simulink model "deep_bram"  (R2016b)
settings: Solver=VariableStepAuto  StartTime=0.0  StopTime=1000  RelTol=1e-3
libraries: xbsIndex_r4 x1049, casper_library_misc x1
(part 2 of 7)

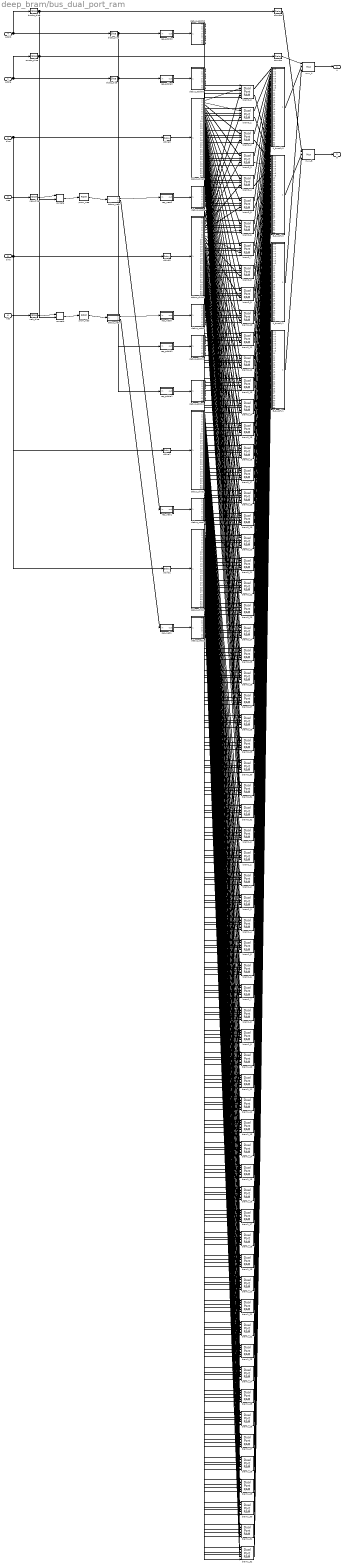
== system deep_bram/bus_dual_port_ram ==
  addra : Inport
  dina : Inport  Port=2
  wea : Inport  Port=3
  addrb : Inport  Port=4
  dinb : Inport  Port=5
  web : Inport  Port=6
  A_bussify0 : Subsystem  AncestorBlock=casper_library_flow_control/bus_create  mask(bus_create){inputNum=33}
      mask prompts: inputNum "Number of inputs:"
      mask init:
      | bus_create_init(gcb,...
      |     'inputNum', inputNum);
  A_bussify1 : Subsystem  AncestorBlock=casper_library_flow_control/bus_create  mask(bus_create){inputNum=33}
      mask prompts: inputNum "Number of inputs:"
      mask init:
      | bus_create_init(gcb,...
      |     'inputNum', inputNum);
  B_bussify0 : Subsystem  AncestorBlock=casper_library_flow_control/bus_create  mask(bus_create){inputNum=33}
      mask prompts: inputNum "Number of inputs:"
      mask init:
      | bus_create_init(gcb,...
      |     'inputNum', inputNum);
  B_bussify1 : Subsystem  AncestorBlock=casper_library_flow_control/bus_create  mask(bus_create){inputNum=33}
      mask prompts: inputNum "Number of inputs:"
      mask init:
      | bus_create_init(gcb,...
      |     'inputNum', inputNum);
  alsbs_slice : xbsIndex_r4/Slice  nbits=17  boolean_output=off  mode=Lower Bit Location + Width  bit1=0  base1=LSB of Input  bit0=0  base0=LSB of Input  dbl_ovrd=off  block_type=slice
  amsbs_slice : xbsIndex_r4/Slice  nbits=1  boolean_output=off  mode=Upper Bit Location + Width  bit1=0  base1=MSB of Input  bit0=0  base0=LSB of Input  dbl_ovrd=off  block_type=slice
  blsbs_slice : xbsIndex_r4/Slice  nbits=14  boolean_output=off  mode=Lower Bit Location + Width  bit1=0  base1=LSB of Input  bit0=0  base0=LSB of Input  dbl_ovrd=off  block_type=slice
  bmsbs_slice : xbsIndex_r4/Slice  nbits=1  boolean_output=off  mode=Upper Bit Location + Width  bit1=0  base1=MSB of Input  bit0=0  base0=LSB of Input  dbl_ovrd=off  block_type=slice
  bram0_{0..32} (33 alike) : xbsIndex_r4/Dual Port RAM  depth=131072  initVector=getfield(get_param(gcb, 'UserData'), 'initVector')  distributed_mem=Block RAM  init_a=0  init_b=0  rst_a=off  rst_b=off  en_a=off  en_b=off  latency=3  write_mode_A=Read Before Write  write_mode_B=Read Before Write  optimize=Speed  dbl_ovrd=off  block_type=dpram
  bram1_{0..32} (33 alike) : xbsIndex_r4/Dual Port RAM  depth=131072  initVector=getfield(get_param(gcb, 'UserData'), 'initVector')  distributed_mem=Block RAM  init_a=0  init_b=0  rst_a=off  rst_b=off  en_a=off  en_b=off  latency=3  write_mode_A=Read Before Write  write_mode_B=Read Before Write  optimize=Speed  dbl_ovrd=off  block_type=dpram
  concata : xbsIndex_r4/Concat  num_inputs=2  dbl_ovrd=off  block_type=concat
  concatb : xbsIndex_r4/Concat  num_inputs=2  dbl_ovrd=off  block_type=concat
  damsbs : xbsIndex_r4/Delay  rst=off  infoeditControl=Selection of Reset will increase slice count due to use of real FFs and instead of SRLs  en=off  latency=2+3  reg_retiming=off  dbl_ovrd=off  block_type=delay
      settings: infoedit=Hardware notes: A delay line is a chain, each link of which is an SRL16 or SRL32 followed by a flip-flop.
  dbmsbs : xbsIndex_r4/Delay  rst=off  infoeditControl=Selection of Reset will increase slice count due to use of real FFs and instead of SRLs  en=off  latency=2+3  reg_retiming=off  dbl_ovrd=off  block_type=delay
      settings: infoedit=Hardware notes: A delay line is a chain, each link of which is an SRL16 or SRL32 followed by a flip-flop.
  ddina0 : xbsIndex_r4/Delay  rst=off  infoeditControl=Selection of Reset will increase slice count due to use of real FFs and instead of SRLs  en=off  latency=2  reg_retiming=off  dbl_ovrd=off  block_type=delay
      settings: infoedit=Hardware notes: A delay line is a chain, each link of which is an SRL16 or SRL32 followed by a flip-flop.
  ddina1 : xbsIndex_r4/Delay  rst=off  infoeditControl=Selection of Reset will increase slice count due to use of real FFs and instead of SRLs  en=off  latency=2  reg_retiming=off  dbl_ovrd=off  block_type=delay
      settings: infoedit=Hardware notes: A delay line is a chain, each link of which is an SRL16 or SRL32 followed by a flip-flop.
  ddinb0 : xbsIndex_r4/Delay  rst=off  infoeditControl=Selection of Reset will increase slice count due to use of real FFs and instead of SRLs  en=off  latency=2  reg_retiming=off  dbl_ovrd=off  block_type=delay
      settings: infoedit=Hardware notes: A delay line is a chain, each link of which is an SRL16 or SRL32 followed by a flip-flop.
  ddinb1 : xbsIndex_r4/Delay  rst=off  infoeditControl=Selection of Reset will increase slice count due to use of real FFs and instead of SRLs  en=off  latency=2  reg_retiming=off  dbl_ovrd=off  block_type=delay
      settings: infoedit=Hardware notes: A delay line is a chain, each link of which is an SRL16 or SRL32 followed by a flip-flop.
  debus_addra0 : Subsystem  AncestorBlock=casper_library_flow_control/bus_expand  mask(bus_expand){mode=divisions of equal size, outputNum=9, outputWidth=[17 17 17 17 17 17 17 17 17], outputBinaryPt=[0 0 0 0 0 0 0 0 0], outputArithmeticType=[0 0 0 0 0 0 0 0 0], show_format=on, outputToWorkspace=off, variablePrefix=, outputToModelAsWell=on}
      mask prompts: outputNum "Number of outputs:"; outputWidth "Output width:"; outputBinaryPt "Output binary point position:"; outputArithmeticType "Output arithmetic type (ufix=0, fix=1, bool=2):"; show_format "Print format string?"; outputToWorkspace "Output to workspace?"; variablePrefix "Variable name prefix:"; outputToModelAsWell "Output to model as well?"
      mask help:
      | Expands a 'bus' made using a bus_create or Xilinx
      | concat block.
      | The input will be divided into the specified number
      | of outputs with the specified arithmetic types.
      | Divisions are made from most significant bit.
      mask init: same as deep_bram/bus_expand
      settings: AttributesFormatString=9 outputs: uf17.0,uf17.0,uf17.0,uf17.0,uf17.0,uf17.0,uf17.0,uf17.0,uf17.0,
      mask TypeOptions mode: divisions of equal size | divisions of arbitrary size
      mask Callback mode: bus_expand_callback();
      mask Callback outputWidth: bus_expand_callback();
      mask Callback outputToWorkspace: bus_expand_callback();
  debus_addra1 : Subsystem  AncestorBlock=casper_library_flow_control/bus_expand  mask(bus_expand){mode=divisions of equal size, outputNum=9, outputWidth=[17 17 17 17 17 17 17 17 17], outputBinaryPt=[0 0 0 0 0 0 0 0 0], outputArithmeticType=[0 0 0 0 0 0 0 0 0], show_format=on, outputToWorkspace=off, variablePrefix=, outputToModelAsWell=on}
      mask prompts: outputNum "Number of outputs:"; outputWidth "Output width:"; outputBinaryPt "Output binary point position:"; outputArithmeticType "Output arithmetic type (ufix=0, fix=1, bool=2):"; show_format "Print format string?"; outputToWorkspace "Output to workspace?"; variablePrefix "Variable name prefix:"; outputToModelAsWell "Output to model as well?"
      mask help:
      | Expands a 'bus' made using a bus_create or Xilinx
      | concat block.
      | The input will be divided into the specified number
      | of outputs with the specified arithmetic types.
      | Divisions are made from most significant bit.
      mask init: same as deep_bram/bus_expand
      settings: AttributesFormatString=9 outputs: uf17.0,uf17.0,uf17.0,uf17.0,uf17.0,uf17.0,uf17.0,uf17.0,uf17.0,
      mask TypeOptions mode: divisions of equal size | divisions of arbitrary size
      mask Callback mode: bus_expand_callback();
      mask Callback outputWidth: bus_expand_callback();
      mask Callback outputToWorkspace: bus_expand_callback();
  debus_addrb0 : Subsystem  AncestorBlock=casper_library_flow_control/bus_expand  mask(bus_expand){mode=divisions of equal size, outputNum=9, outputWidth=[14 14 14 14 14 14 14 14 14], outputBinaryPt=[0 0 0 0 0 0 0 0 0], outputArithmeticType=[0 0 0 0 0 0 0 0 0], show_format=on, outputToWorkspace=off, variablePrefix=, outputToModelAsWell=on}
      mask prompts: outputNum "Number of outputs:"; outputWidth "Output width:"; outputBinaryPt "Output binary point position:"; outputArithmeticType "Output arithmetic type (ufix=0, fix=1, bool=2):"; show_format "Print format string?"; outputToWorkspace "Output to workspace?"; variablePrefix "Variable name prefix:"; outputToModelAsWell "Output to model as well?"
      mask help:
      | Expands a 'bus' made using a bus_create or Xilinx
      | concat block.
      | The input will be divided into the specified number
      | of outputs with the specified arithmetic types.
      | Divisions are made from most significant bit.
      mask init: same as deep_bram/bus_expand
      settings: AttributesFormatString=9 outputs: uf14.0,uf14.0,uf14.0,uf14.0,uf14.0,uf14.0,uf14.0,uf14.0,uf14.0,
      mask TypeOptions mode: divisions of equal size | divisions of arbitrary size
      mask Callback mode: bus_expand_callback();
      mask Callback outputWidth: bus_expand_callback();
      mask Callback outputToWorkspace: bus_expand_callback();
  debus_addrb1 : Subsystem  AncestorBlock=casper_library_flow_control/bus_expand  mask(bus_expand){mode=divisions of equal size, outputNum=9, outputWidth=[14 14 14 14 14 14 14 14 14], outputBinaryPt=[0 0 0 0 0 0 0 0 0], outputArithmeticType=[0 0 0 0 0 0 0 0 0], show_format=on, outputToWorkspace=off, variablePrefix=, outputToModelAsWell=on}
      mask prompts: outputNum "Number of outputs:"; outputWidth "Output width:"; outputBinaryPt "Output binary point position:"; outputArithmeticType "Output arithmetic type (ufix=0, fix=1, bool=2):"; show_format "Print format string?"; outputToWorkspace "Output to workspace?"; variablePrefix "Variable name prefix:"; outputToModelAsWell "Output to model as well?"
      mask help:
      | Expands a 'bus' made using a bus_create or Xilinx
      | concat block.
      | The input will be divided into the specified number
      | of outputs with the specified arithmetic types.
      | Divisions are made from most significant bit.
      mask init: same as deep_bram/bus_expand
      settings: AttributesFormatString=9 outputs: uf14.0,uf14.0,uf14.0,uf14.0,uf14.0,uf14.0,uf14.0,uf14.0,uf14.0,
      mask TypeOptions mode: divisions of equal size | divisions of arbitrary size
      mask Callback mode: bus_expand_callback();
      mask Callback outputWidth: bus_expand_callback();
      mask Callback outputToWorkspace: bus_expand_callback();
  debus_dina0 : Subsystem  AncestorBlock=casper_library_flow_control/bus_expand  mask(bus_expand){mode=divisions of arbitrary size, outputNum=1, outputWidth=[1 1 1 1 1 1 1 1 1 1 1 1 1 1 1 1 1 1 1 1 1 1 1 1 1 1 1 1 1 1 1 1 1], outputBinaryPt=[0 0 0 0 0 0 0 0 0 0 0 0 0 0 0 0 0 0 0 0 0 0 0 0 0 0 0 0 0 0 0 0 0], outputArithmeticType=[0 0 0 0 0 0 0 0 0 0 0 0 0 0 0 0 0 0 0 0 0 0 0 0 0 0 0 0 0 0 0 0 0], show_format=on, outputToWorkspace=off, variablePrefix=, outputToModelAsWell=on}
      mask prompts: outputNum "Number of outputs:"; outputWidth "Output width [msb ... lsb]:"; outputBinaryPt "Output binary point position [msb ... lsb]:"; outputArithmeticType "Output arithmetic type (ufix=0, fix=1, bool=2) [msb ... lsb]:"; show_format "Print format string?"; outputToWorkspace "Output to workspace?"; variablePrefix "Variable name prefix:"; outputToModelAsWell "Output to model as well?"
      mask help:
      | Expands a 'bus' made using a bus_create or Xilinx
      | concat block.
      | The input will be divided into the specified number
      | of outputs with the specified arithmetic types.
      | Divisions are made from most significant bit.
      mask init: same as deep_bram/bus_expand
      settings: AttributesFormatString=33 outputs: uf1.0,uf1.0,uf1.0,uf1.0,uf1.0,uf1.0,uf1.0,uf1.0,uf1.0,uf1.0,uf1.0,uf1.0,uf1.0,uf1.0,uf1.0,uf1.0,uf1.0,uf1.0,uf1.0,uf1.0,uf1.0,uf1.0,uf1.0,uf1.0,uf1.0,uf1.0,uf1.0,uf1.0,uf1.0,uf1.0,uf1.0,uf1.0,uf1.0,
      mask TypeOptions mode: divisions of equal size | divisions of arbitrary size
      mask Callback mode: bus_expand_callback();
      mask Callback outputWidth: bus_expand_callback();
      mask Callback outputToWorkspace: bus_expand_callback();
  debus_dina1 : Subsystem  AncestorBlock=casper_library_flow_control/bus_expand  mask(bus_expand){mode=divisions of arbitrary size, outputNum=1, outputWidth=[1 1 1 1 1 1 1 1 1 1 1 1 1 1 1 1 1 1 1 1 1 1 1 1 1 1 1 1 1 1 1 1 1], outputBinaryPt=[0 0 0 0 0 0 0 0 0 0 0 0 0 0 0 0 0 0 0 0 0 0 0 0 0 0 0 0 0 0 0 0 0], outputArithmeticType=[0 0 0 0 0 0 0 0 0 0 0 0 0 0 0 0 0 0 0 0 0 0 0 0 0 0 0 0 0 0 0 0 0], show_format=on, outputToWorkspace=off, variablePrefix=, outputToModelAsWell=on}
      mask prompts: outputNum "Number of outputs:"; outputWidth "Output width [msb ... lsb]:"; outputBinaryPt "Output binary point position [msb ... lsb]:"; outputArithmeticType "Output arithmetic type (ufix=0, fix=1, bool=2) [msb ... lsb]:"; show_format "Print format string?"; outputToWorkspace "Output to workspace?"; variablePrefix "Variable name prefix:"; outputToModelAsWell "Output to model as well?"
      mask help:
      | Expands a 'bus' made using a bus_create or Xilinx
      | concat block.
      | The input will be divided into the specified number
      | of outputs with the specified arithmetic types.
      | Divisions are made from most significant bit.
      mask init: same as deep_bram/bus_expand
      settings: AttributesFormatString=33 outputs: uf1.0,uf1.0,uf1.0,uf1.0,uf1.0,uf1.0,uf1.0,uf1.0,uf1.0,uf1.0,uf1.0,uf1.0,uf1.0,uf1.0,uf1.0,uf1.0,uf1.0,uf1.0,uf1.0,uf1.0,uf1.0,uf1.0,uf1.0,uf1.0,uf1.0,uf1.0,uf1.0,uf1.0,uf1.0,uf1.0,uf1.0,uf1.0,uf1.0,
      mask TypeOptions mode: divisions of equal size | divisions of arbitrary size
      mask Callback mode: bus_expand_callback();
      mask Callback outputWidth: bus_expand_callback();
      mask Callback outputToWorkspace: bus_expand_callback();
  debus_dinb0 : Subsystem  AncestorBlock=casper_library_flow_control/bus_expand  mask(bus_expand){mode=divisions of arbitrary size, outputNum=1, outputWidth=[8 8 8 8 8 8 8 8 8 8 8 8 8 8 8 8 8 8 8 8 8 8 8 8 8 8 8 8 8 8 8 8 8], outputBinaryPt=[0 0 0 0 0 0 0 0 0 0 0 0 0 0 0 0 0 0 0 0 0 0 0 0 0 0 0 0 0 0 0 0 0], outputArithmeticType=[0 0 0 0 0 0 0 0 0 0 0 0 0 0 0 0 0 0 0 0 0 0 0 0 0 0 0 0 0 0 0 0 0], show_format=on, outputToWorkspace=off, variablePrefix=, outputToModelAsWell=on}
      mask prompts: outputNum "Number of outputs:"; outputWidth "Output width [msb ... lsb]:"; outputBinaryPt "Output binary point position [msb ... lsb]:"; outputArithmeticType "Output arithmetic type (ufix=0, fix=1, bool=2) [msb ... lsb]:"; show_format "Print format string?"; outputToWorkspace "Output to workspace?"; variablePrefix "Variable name prefix:"; outputToModelAsWell "Output to model as well?"
      mask help:
      | Expands a 'bus' made using a bus_create or Xilinx
      | concat block.
      | The input will be divided into the specified number
      | of outputs with the specified arithmetic types.
      | Divisions are made from most significant bit.
      mask init: same as deep_bram/bus_expand
      settings: AttributesFormatString=33 outputs: uf8.0,uf8.0,uf8.0,uf8.0,uf8.0,uf8.0,uf8.0,uf8.0,uf8.0,uf8.0,uf8.0,uf8.0,uf8.0,uf8.0,uf8.0,uf8.0,uf8.0,uf8.0,uf8.0,uf8.0,uf8.0,uf8.0,uf8.0,uf8.0,uf8.0,uf8.0,uf8.0,uf8.0,uf8.0,uf8.0,uf8.0,uf8.0,uf8.0,
      mask TypeOptions mode: divisions of equal size | divisions of arbitrary size
      mask Callback mode: bus_expand_callback();
      mask Callback outputWidth: bus_expand_callback();
      mask Callback outputToWorkspace: bus_expand_callback();
  debus_dinb1 : Subsystem  AncestorBlock=casper_library_flow_control/bus_expand  mask(bus_expand){mode=divisions of arbitrary size, outputNum=1, outputWidth=[8 8 8 8 8 8 8 8 8 8 8 8 8 8 8 8 8 8 8 8 8 8 8 8 8 8 8 8 8 8 8 8 8], outputBinaryPt=[0 0 0 0 0 0 0 0 0 0 0 0 0 0 0 0 0 0 0 0 0 0 0 0 0 0 0 0 0 0 0 0 0], outputArithmeticType=[0 0 0 0 0 0 0 0 0 0 0 0 0 0 0 0 0 0 0 0 0 0 0 0 0 0 0 0 0 0 0 0 0], show_format=on, outputToWorkspace=off, variablePrefix=, outputToModelAsWell=on}
      mask prompts: outputNum "Number of outputs:"; outputWidth "Output width [msb ... lsb]:"; outputBinaryPt "Output binary point position [msb ... lsb]:"; outputArithmeticType "Output arithmetic type (ufix=0, fix=1, bool=2) [msb ... lsb]:"; show_format "Print format string?"; outputToWorkspace "Output to workspace?"; variablePrefix "Variable name prefix:"; outputToModelAsWell "Output to model as well?"
      mask help:
      | Expands a 'bus' made using a bus_create or Xilinx
      | concat block.
      | The input will be divided into the specified number
      | of outputs with the specified arithmetic types.
      | Divisions are made from most significant bit.
      mask init: same as deep_bram/bus_expand
      settings: AttributesFormatString=33 outputs: uf8.0,uf8.0,uf8.0,uf8.0,uf8.0,uf8.0,uf8.0,uf8.0,uf8.0,uf8.0,uf8.0,uf8.0,uf8.0,uf8.0,uf8.0,uf8.0,uf8.0,uf8.0,uf8.0,uf8.0,uf8.0,uf8.0,uf8.0,uf8.0,uf8.0,uf8.0,uf8.0,uf8.0,uf8.0,uf8.0,uf8.0,uf8.0,uf8.0,
      mask TypeOptions mode: divisions of equal size | divisions of arbitrary size
      mask Callback mode: bus_expand_callback();
      mask Callback outputWidth: bus_expand_callback();
      mask Callback outputToWorkspace: bus_expand_callback();
  debus_wea : Subsystem  AncestorBlock=casper_library_flow_control/bus_expand  mask(bus_expand){mode=divisions of equal size, outputNum=2, outputWidth=[1 1], outputBinaryPt=[0 0], outputArithmeticType=[2 2], show_format=on, outputToWorkspace=off, variablePrefix=, outputToModelAsWell=on}
      mask prompts: outputNum "Number of outputs:"; outputWidth "Output width:"; outputBinaryPt "Output binary point position:"; outputArithmeticType "Output arithmetic type (ufix=0, fix=1, bool=2):"; show_format "Print format string?"; outputToWorkspace "Output to workspace?"; variablePrefix "Variable name prefix:"; outputToModelAsWell "Output to model as well?"
      mask help:
      | Expands a 'bus' made using a bus_create or Xilinx
      | concat block.
      | The input will be divided into the specified number
      | of outputs with the specified arithmetic types.
      | Divisions are made from most significant bit.
      mask init: same as deep_bram/bus_expand
      settings: AttributesFormatString=2 outputs: b,b,
      mask TypeOptions mode: divisions of equal size | divisions of arbitrary size
      mask Callback mode: bus_expand_callback();
      mask Callback outputWidth: bus_expand_callback();
      mask Callback outputToWorkspace: bus_expand_callback();
  debus_wea0 : Subsystem  AncestorBlock=casper_library_flow_control/bus_expand  mask(bus_expand){mode=divisions of equal size, outputNum=9, outputWidth=[1 1 1 1 1 1 1 1 1], outputBinaryPt=[0 0 0 0 0 0 0 0 0], outputArithmeticType=[2 2 2 2 2 2 2 2 2], show_format=on, outputToWorkspace=off, variablePrefix=, outputToModelAsWell=on}
      mask prompts: outputNum "Number of outputs:"; outputWidth "Output width:"; outputBinaryPt "Output binary point position:"; outputArithmeticType "Output arithmetic type (ufix=0, fix=1, bool=2):"; show_format "Print format string?"; outputToWorkspace "Output to workspace?"; variablePrefix "Variable name prefix:"; outputToModelAsWell "Output to model as well?"
      mask help:
      | Expands a 'bus' made using a bus_create or Xilinx
      | concat block.
      | The input will be divided into the specified number
      | of outputs with the specified arithmetic types.
      | Divisions are made from most significant bit.
      mask init: same as deep_bram/bus_expand
      settings: AttributesFormatString=9 outputs: b,b,b,b,b,b,b,b,b,
      mask TypeOptions mode: divisions of equal size | divisions of arbitrary size
      mask Callback mode: bus_expand_callback();
      mask Callback outputWidth: bus_expand_callback();
      mask Callback outputToWorkspace: bus_expand_callback();
  debus_wea1 : Subsystem  AncestorBlock=casper_library_flow_control/bus_expand  mask(bus_expand){mode=divisions of equal size, outputNum=9, outputWidth=[1 1 1 1 1 1 1 1 1], outputBinaryPt=[0 0 0 0 0 0 0 0 0], outputArithmeticType=[2 2 2 2 2 2 2 2 2], show_format=on, outputToWorkspace=off, variablePrefix=, outputToModelAsWell=on}
      mask prompts: outputNum "Number of outputs:"; outputWidth "Output width:"; outputBinaryPt "Output binary point position:"; outputArithmeticType "Output arithmetic type (ufix=0, fix=1, bool=2):"; show_format "Print format string?"; outputToWorkspace "Output to workspace?"; variablePrefix "Variable name prefix:"; outputToModelAsWell "Output to model as well?"
      mask help:
      | Expands a 'bus' made using a bus_create or Xilinx
      | concat block.
      | The input will be divided into the specified number
      | of outputs with the specified arithmetic types.
      | Divisions are made from most significant bit.
      mask init: same as deep_bram/bus_expand
      settings: AttributesFormatString=9 outputs: b,b,b,b,b,b,b,b,b,
      mask TypeOptions mode: divisions of equal size | divisions of arbitrary size
      mask Callback mode: bus_expand_callback();
      mask Callback outputWidth: bus_expand_callback();
      mask Callback outputToWorkspace: bus_expand_callback();
  debus_web : Subsystem  AncestorBlock=casper_library_flow_control/bus_expand  mask(bus_expand){mode=divisions of equal size, outputNum=2, outputWidth=[1 1], outputBinaryPt=[0 0], outputArithmeticType=[2 2], show_format=on, outputToWorkspace=off, variablePrefix=, outputToModelAsWell=on}
      mask prompts: outputNum "Number of outputs:"; outputWidth "Output width:"; outputBinaryPt "Output binary point position:"; outputArithmeticType "Output arithmetic type (ufix=0, fix=1, bool=2):"; show_format "Print format string?"; outputToWorkspace "Output to workspace?"; variablePrefix "Variable name prefix:"; outputToModelAsWell "Output to model as well?"
      mask help:
      | Expands a 'bus' made using a bus_create or Xilinx
      | concat block.
      | The input will be divided into the specified number
      | of outputs with the specified arithmetic types.
      | Divisions are made from most significant bit.
      mask init: same as deep_bram/bus_expand
      settings: AttributesFormatString=2 outputs: b,b,
      mask TypeOptions mode: divisions of equal size | divisions of arbitrary size
      mask Callback mode: bus_expand_callback();
      mask Callback outputWidth: bus_expand_callback();
      mask Callback outputToWorkspace: bus_expand_callback();
  debus_web0 : Subsystem  AncestorBlock=casper_library_flow_control/bus_expand  mask(bus_expand){mode=divisions of equal size, outputNum=9, outputWidth=[1 1 1 1 1 1 1 1 1], outputBinaryPt=[0 0 0 0 0 0 0 0 0], outputArithmeticType=[2 2 2 2 2 2 2 2 2], show_format=on, outputToWorkspace=off, variablePrefix=, outputToModelAsWell=on}
      mask prompts: outputNum "Number of outputs:"; outputWidth "Output width:"; outputBinaryPt "Output binary point position:"; outputArithmeticType "Output arithmetic type (ufix=0, fix=1, bool=2):"; show_format "Print format string?"; outputToWorkspace "Output to workspace?"; variablePrefix "Variable name prefix:"; outputToModelAsWell "Output to model as well?"
      mask help:
      | Expands a 'bus' made using a bus_create or Xilinx
      | concat block.
      | The input will be divided into the specified number
      | of outputs with the specified arithmetic types.
      | Divisions are made from most significant bit.
      mask init: same as deep_bram/bus_expand
      settings: AttributesFormatString=9 outputs: b,b,b,b,b,b,b,b,b,
      mask TypeOptions mode: divisions of equal size | divisions of arbitrary size
      mask Callback mode: bus_expand_callback();
      mask Callback outputWidth: bus_expand_callback();
      mask Callback outputToWorkspace: bus_expand_callback();
  debus_web1 : Subsystem  AncestorBlock=casper_library_flow_control/bus_expand  mask(bus_expand){mode=divisions of equal size, outputNum=9, outputWidth=[1 1 1 1 1 1 1 1 1], outputBinaryPt=[0 0 0 0 0 0 0 0 0], outputArithmeticType=[2 2 2 2 2 2 2 2 2], show_format=on, outputToWorkspace=off, variablePrefix=, outputToModelAsWell=on}
      mask prompts: outputNum "Number of outputs:"; outputWidth "Output width:"; outputBinaryPt "Output binary point position:"; outputArithmeticType "Output arithmetic type (ufix=0, fix=1, bool=2):"; show_format "Print format string?"; outputToWorkspace "Output to workspace?"; variablePrefix "Variable name prefix:"; outputToModelAsWell "Output to model as well?"
      mask help:
      | Expands a 'bus' made using a bus_create or Xilinx
      | concat block.
      | The input will be divided into the specified number
      | of outputs with the specified arithmetic types.
      | Divisions are made from most significant bit.
      mask init: same as deep_bram/bus_expand
      settings: AttributesFormatString=9 outputs: b,b,b,b,b,b,b,b,b,
      mask TypeOptions mode: divisions of equal size | divisions of arbitrary size
      mask Callback mode: bus_expand_callback();
      mask Callback outputWidth: bus_expand_callback();
      mask Callback outputToWorkspace: bus_expand_callback();
  mux_A : xbsIndex_r4/Mux  inputs=2  en=off  latency=0  precision=Full  arith_type=Unsigned  n_bits=16  bin_pt=14  quantization=Truncate  overflow=Wrap  dbl_ovrd=off  block_type=mux
  mux_B : xbsIndex_r4/Mux  inputs=2  en=off  latency=0  precision=Full  arith_type=Unsigned  n_bits=16  bin_pt=14  quantization=Truncate  overflow=Wrap  dbl_ovrd=off  block_type=mux
  prom_wea : xbsIndex_r4/ROM  depth=4  initVector=[0 0 2 1]  distributed_mem=Distributed memory  rst=off  init_reg=0  en=off  latency=0  gui_display_data_type=Fixed-point  arith_type=Unsigned  n_bits=2  bin_pt=0  preci_type=Single  exp_width=8  frac_width=24  optimize=Area  use_rpm=on  dbl_ovrd=off  block_type=sprom
  prom_web : xbsIndex_r4/ROM  depth=4  initVector=[0 0 2 1]  distributed_mem=Distributed memory  rst=off  init_reg=0  en=off  latency=0  gui_display_data_type=Fixed-point  arith_type=Unsigned  n_bits=2  bin_pt=0  preci_type=Single  exp_width=8  frac_width=24  optimize=Area  use_rpm=on  dbl_ovrd=off  block_type=sprom
  rep_addra0 : Subsystem  AncestorBlock=casper_library_bus/bus_replicate  mask(bus_replicate){replication=9, latency=2, misc=off, implementation=core}
      mask prompts: replication "replication factor"; misc "misc support"; implementation "delay implementation"
      mask help: Output bus formed by replicating input bus a number of times
      mask init:
      | bus_replicate_init(gcb, ...
      |     'replication', replication, ...
      |     'latency', latency, ...
      |     'implementation', implementation, ...
      |     'misc', misc);
      mask TypeOptions implementation: core | behavioral
  rep_addra1 : Subsystem  AncestorBlock=casper_library_bus/bus_replicate  mask(bus_replicate){replication=9, latency=2, misc=off, implementation=core}
      mask prompts: replication "replication factor"; misc "misc support"; implementation "delay implementation"
      mask help: Output bus formed by replicating input bus a number of times
      mask init:
      | bus_replicate_init(gcb, ...
      |     'replication', replication, ...
      |     'latency', latency, ...
      |     'implementation', implementation, ...
      |     'misc', misc);
      mask TypeOptions implementation: core | behavioral
  rep_addrb0 : Subsystem  AncestorBlock=casper_library_bus/bus_replicate  mask(bus_replicate){replication=9, latency=2, misc=off, implementation=core}
      mask prompts: replication "replication factor"; misc "misc support"; implementation "delay implementation"
      mask help: Output bus formed by replicating input bus a number of times
      mask init:
      | bus_replicate_init(gcb, ...
      |     'replication', replication, ...
      |     'latency', latency, ...
      |     'implementation', implementation, ...
      |     'misc', misc);
      mask TypeOptions implementation: core | behavioral
  rep_addrb1 : Subsystem  AncestorBlock=casper_library_bus/bus_replicate  mask(bus_replicate){replication=9, latency=2, misc=off, implementation=core}
      mask prompts: replication "replication factor"; misc "misc support"; implementation "delay implementation"
      mask help: Output bus formed by replicating input bus a number of times
      mask init:
      | bus_replicate_init(gcb, ...
      |     'replication', replication, ...
      |     'latency', latency, ...
      |     'implementation', implementation, ...
      |     'misc', misc);
      mask TypeOptions implementation: core | behavioral
  rep_wea0 : Subsystem  AncestorBlock=casper_library_bus/bus_replicate  mask(bus_replicate){replication=9, latency=2, misc=off, implementation=core}
      mask prompts: replication "replication factor"; misc "misc support"; implementation "delay implementation"
      mask help: Output bus formed by replicating input bus a number of times
      mask init:
      | bus_replicate_init(gcb, ...
      |     'replication', replication, ...
      |     'latency', latency, ...
      |     'implementation', implementation, ...
      |     'misc', misc);
      mask TypeOptions implementation: core | behavioral
  rep_wea1 : Subsystem  AncestorBlock=casper_library_bus/bus_replicate  mask(bus_replicate){replication=9, latency=2, misc=off, implementation=core}
      mask prompts: replication "replication factor"; misc "misc support"; implementation "delay implementation"
      mask help: Output bus formed by replicating input bus a number of times
      mask init:
      | bus_replicate_init(gcb, ...
      |     'replication', replication, ...
      |     'latency', latency, ...
      |     'implementation', implementation, ...
      |     'misc', misc);
      mask TypeOptions implementation: core | behavioral
  rep_web0 : Subsystem  AncestorBlock=casper_library_bus/bus_replicate  mask(bus_replicate){replication=9, latency=2, misc=off, implementation=core}
      mask prompts: replication "replication factor"; misc "misc support"; implementation "delay implementation"
      mask help: Output bus formed by replicating input bus a number of times
      mask init:
      | bus_replicate_init(gcb, ...
      |     'replication', replication, ...
      |     'latency', latency, ...
      |     'implementation', implementation, ...
      |     'misc', misc);
      mask TypeOptions implementation: core | behavioral
  rep_web1 : Subsystem  AncestorBlock=casper_library_bus/bus_replicate  mask(bus_replicate){replication=9, latency=2, misc=off, implementation=core}
      mask prompts: replication "replication factor"; misc "misc support"; implementation "delay implementation"
      mask help: Output bus formed by replicating input bus a number of times
      mask init:
      | bus_replicate_init(gcb, ...
      |     'replication', replication, ...
      |     'latency', latency, ...
      |     'implementation', implementation, ...
      |     'misc', misc);
      mask TypeOptions implementation: core | behavioral
  wea_slice : xbsIndex_r4/Slice  nbits=1  boolean_output=off  mode=Upper Bit Location + Width  bit1=0  base1=MSB of Input  bit0=0  base0=LSB of Input  dbl_ovrd=off  block_type=slice
  web_slice : xbsIndex_r4/Slice  nbits=1  boolean_output=off  mode=Upper Bit Location + Width  bit1=0  base1=MSB of Input  bit0=0  base0=LSB of Input  dbl_ovrd=off  block_type=slice
  A : Outport
  B : Outport  Port=2
  wires:
  addrb/1 -> bmsbs_slice/1, blsbs_slice/1
  addra/1 -> amsbs_slice/1, alsbs_slice/1
  wea/1 -> wea_slice/1
  web/1 -> web_slice/1
  wea_slice/1 -> concata/1
  amsbs_slice/1 -> concata/2, damsbs/1
  web_slice/1 -> concatb/1
  bmsbs_slice/1 -> concatb/2, dbmsbs/1
  concata/1 -> prom_wea/1
  concatb/1 -> prom_web/1
  prom_wea/1 -> debus_wea/1(bus_in)
  prom_web/1 -> debus_web/1(bus_in)
  blsbs_slice/1 -> rep_addrb0/1(in), rep_addrb1/1(in)
  alsbs_slice/1 -> rep_addra0/1(in), rep_addra1/1(in)
  dina/1 -> ddina0/1, ddina1/1
  debus_wea/1(msb_out2) -> rep_wea0/1(in)
  dinb/1 -> ddinb0/1, ddinb1/1
  debus_web/1(msb_out2) -> rep_web0/1(in)
  debus_wea/2(lsb_out1) -> rep_wea1/1(in)
  debus_web/2(lsb_out1) -> rep_web1/1(in)
  rep_addrb0/1(out) -> debus_addrb0/1(bus_in)
  rep_addra0/1(out) -> debus_addra0/1(bus_in)
  ddina0/1 -> debus_dina0/1(bus_in)
  rep_wea0/1(out) -> debus_wea0/1(bus_in)
  ddinb0/1 -> debus_dinb0/1(bus_in)
  rep_web0/1(out) -> debus_web0/1(bus_in)
  rep_addrb1/1(out) -> debus_addrb1/1(bus_in)
  rep_addra1/1(out) -> debus_addra1/1(bus_in)
  ddina1/1 -> debus_dina1/1(bus_in)
  rep_wea1/1(out) -> debus_wea1/1(bus_in)
  ddinb1/1 -> debus_dinb1/1(bus_in)
  rep_web1/1(out) -> debus_web1/1(bus_in)
  debus_addra0/1(msb_out9) -> bram0_0/1, bram0_9/1, bram0_18/1, bram0_27/1
  debus_dina0/1(msb_out33) -> bram0_0/2
  debus_wea0/1(msb_out9) -> bram0_0/3, bram0_9/3, bram0_18/3, bram0_27/3
  debus_addrb0/1(msb_out9) -> bram0_0/4, bram0_9/4, bram0_18/4, bram0_27/4
  debus_dinb0/1(msb_out33) -> bram0_0/5
  debus_web0/1(msb_out9) -> bram0_0/6, bram0_9/6, bram0_18/6, bram0_27/6
  debus_addra0/2(out8) -> bram0_1/1, bram0_10/1, bram0_19/1, bram0_28/1
  debus_dina0/2(out32) -> bram0_1/2
  debus_wea0/2(out8) -> bram0_1/3, bram0_10/3, bram0_19/3, bram0_28/3
  debus_addrb0/2(out8) -> bram0_1/4, bram0_10/4, bram0_19/4, bram0_28/4
  debus_dinb0/2(out32) -> bram0_1/5
  debus_web0/2(out8) -> bram0_1/6, bram0_10/6, bram0_19/6, bram0_28/6
  debus_addra0/3(out7) -> bram0_2/1, bram0_11/1, bram0_20/1, bram0_29/1
  debus_dina0/3(out31) -> bram0_2/2
  debus_wea0/3(out7) -> bram0_2/3, bram0_11/3, bram0_20/3, bram0_29/3
  debus_addrb0/3(out7) -> bram0_2/4, bram0_11/4, bram0_20/4, bram0_29/4
  debus_dinb0/3(out31) -> bram0_2/5
  debus_web0/3(out7) -> bram0_2/6, bram0_11/6, bram0_20/6, bram0_29/6
  debus_addra0/4(out6) -> bram0_3/1, bram0_12/1, bram0_21/1, bram0_30/1
  debus_dina0/4(out30) -> bram0_3/2
  debus_wea0/4(out6) -> bram0_3/3, bram0_12/3, bram0_21/3, bram0_30/3
  debus_addrb0/4(out6) -> bram0_3/4, bram0_12/4, bram0_21/4, bram0_30/4
  debus_dinb0/4(out30) -> bram0_3/5
  debus_web0/4(out6) -> bram0_3/6, bram0_12/6, bram0_21/6, bram0_30/6
  debus_addra0/5(out5) -> bram0_4/1, bram0_13/1, bram0_22/1, bram0_31/1
  debus_dina0/5(out29) -> bram0_4/2
  debus_wea0/5(out5) -> bram0_4/3, bram0_13/3, bram0_22/3, bram0_31/3
  debus_addrb0/5(out5) -> bram0_4/4, bram0_13/4, bram0_22/4, bram0_31/4
  debus_dinb0/5(out29) -> bram0_4/5
  debus_web0/5(out5) -> bram0_4/6, bram0_13/6, bram0_22/6, bram0_31/6
  debus_addra0/6(out4) -> bram0_5/1, bram0_14/1, bram0_23/1, bram0_32/1
  debus_dina0/6(out28) -> bram0_5/2
  debus_wea0/6(out4) -> bram0_5/3, bram0_14/3, bram0_23/3, bram0_32/3
  debus_addrb0/6(out4) -> bram0_5/4, bram0_14/4, bram0_23/4, bram0_32/4
  debus_dinb0/6(out28) -> bram0_5/5
  debus_web0/6(out4) -> bram0_5/6, bram0_14/6, bram0_23/6, bram0_32/6
  debus_addra0/7(out3) -> bram0_6/1, bram0_15/1, bram0_24/1
  debus_dina0/7(out27) -> bram0_6/2
  debus_wea0/7(out3) -> bram0_6/3, bram0_15/3, bram0_24/3
  debus_addrb0/7(out3) -> bram0_6/4, bram0_15/4, bram0_24/4
  debus_dinb0/7(out27) -> bram0_6/5
  debus_web0/7(out3) -> bram0_6/6, bram0_15/6, bram0_24/6
  debus_addra0/8(out2) -> bram0_7/1, bram0_16/1, bram0_25/1
  debus_dina0/8(out26) -> bram0_7/2
  debus_wea0/8(out2) -> bram0_7/3, bram0_16/3, bram0_25/3
  debus_addrb0/8(out2) -> bram0_7/4, bram0_16/4, bram0_25/4
  debus_dinb0/8(out26) -> bram0_7/5
  debus_web0/8(out2) -> bram0_7/6, bram0_16/6, bram0_25/6
  debus_addra0/9(lsb_out1) -> bram0_8/1, bram0_17/1, bram0_26/1
  debus_dina0/9(out25) -> bram0_8/2
  debus_wea0/9(lsb_out1) -> bram0_8/3, bram0_17/3, bram0_26/3
  debus_addrb0/9(lsb_out1) -> bram0_8/4, bram0_17/4, bram0_26/4
  debus_dinb0/9(out25) -> bram0_8/5
  debus_web0/9(lsb_out1) -> bram0_8/6, bram0_17/6, bram0_26/6
  debus_dina0/10(out24) -> bram0_9/2
  debus_dinb0/10(out24) -> bram0_9/5
  debus_dina0/11(out23) -> bram0_10/2
  debus_dinb0/11(out23) -> bram0_10/5
  debus_dina0/12(out22) -> bram0_11/2
  debus_dinb0/12(out22) -> bram0_11/5
  debus_dina0/13(out21) -> bram0_12/2
  debus_dinb0/13(out21) -> bram0_12/5
  debus_dina0/14(out20) -> bram0_13/2
  debus_dinb0/14(out20) -> bram0_13/5
  debus_dina0/15(out19) -> bram0_14/2
  debus_dinb0/15(out19) -> bram0_14/5
  debus_dina0/16(out18) -> bram0_15/2
  debus_dinb0/16(out18) -> bram0_15/5
  debus_dina0/17(out17) -> bram0_16/2
  debus_dinb0/17(out17) -> bram0_16/5
  debus_dina0/18(out16) -> bram0_17/2
  debus_dinb0/18(out16) -> bram0_17/5
  debus_dina0/19(out15) -> bram0_18/2
  debus_dinb0/19(out15) -> bram0_18/5
  debus_dina0/20(out14) -> bram0_19/2
  debus_dinb0/20(out14) -> bram0_19/5
  debus_dina0/21(out13) -> bram0_20/2
  debus_dinb0/21(out13) -> bram0_20/5
  debus_dina0/22(out12) -> bram0_21/2
  debus_dinb0/22(out12) -> bram0_21/5
  debus_dina0/23(out11) -> bram0_22/2
  debus_dinb0/23(out11) -> bram0_22/5
  debus_dina0/24(out10) -> bram0_23/2
  debus_dinb0/24(out10) -> bram0_23/5
  debus_dina0/25(out9) -> bram0_24/2
  debus_dinb0/25(out9) -> bram0_24/5
  debus_dina0/26(out8) -> bram0_25/2
  debus_dinb0/26(out8) -> bram0_25/5
  debus_dina0/27(out7) -> bram0_26/2
  debus_dinb0/27(out7) -> bram0_26/5
  debus_dina0/28(out6) -> bram0_27/2
  debus_dinb0/28(out6) -> bram0_27/5
  debus_dina0/29(out5) -> bram0_28/2
  debus_dinb0/29(out5) -> bram0_28/5
  debus_dina0/30(out4) -> bram0_29/2
  debus_dinb0/30(out4) -> bram0_29/5
  debus_dina0/31(out3) -> bram0_30/2
  debus_dinb0/31(out3) -> bram0_30/5
  debus_dina0/32(out2) -> bram0_31/2
  debus_dinb0/32(out2) -> bram0_31/5
  debus_dina0/33(lsb_out1) -> bram0_32/2
  debus_dinb0/33(lsb_out1) -> bram0_32/5
  debus_addra1/1(msb_out9) -> bram1_0/1, bram1_9/1, bram1_18/1, bram1_27/1
  debus_dina1/1(msb_out33) -> bram1_0/2
  debus_wea1/1(msb_out9) -> bram1_0/3, bram1_9/3, bram1_18/3, bram1_27/3
  debus_addrb1/1(msb_out9) -> bram1_0/4, bram1_9/4, bram1_18/4, bram1_27/4
  debus_dinb1/1(msb_out33) -> bram1_0/5
  debus_web1/1(msb_out9) -> bram1_0/6, bram1_9/6, bram1_18/6, bram1_27/6
  debus_addra1/2(out8) -> bram1_1/1, bram1_10/1, bram1_19/1, bram1_28/1
  debus_dina1/2(out32) -> bram1_1/2
  debus_wea1/2(out8) -> bram1_1/3, bram1_10/3, bram1_19/3, bram1_28/3
  debus_addrb1/2(out8) -> bram1_1/4, bram1_10/4, bram1_19/4, bram1_28/4
  debus_dinb1/2(out32) -> bram1_1/5
  debus_web1/2(out8) -> bram1_1/6, bram1_10/6, bram1_19/6, bram1_28/6
  debus_addra1/3(out7) -> bram1_2/1, bram1_11/1, bram1_20/1, bram1_29/1
  debus_dina1/3(out31) -> bram1_2/2
  debus_wea1/3(out7) -> bram1_2/3, bram1_11/3, bram1_20/3, bram1_29/3
  debus_addrb1/3(out7) -> bram1_2/4, bram1_11/4, bram1_20/4, bram1_29/4
  debus_dinb1/3(out31) -> bram1_2/5
  debus_web1/3(out7) -> bram1_2/6, bram1_11/6, bram1_20/6, bram1_29/6
  debus_addra1/4(out6) -> bram1_3/1, bram1_12/1, bram1_21/1, bram1_30/1
  debus_dina1/4(out30) -> bram1_3/2
  debus_wea1/4(out6) -> bram1_3/3, bram1_12/3, bram1_21/3, bram1_30/3
  debus_addrb1/4(out6) -> bram1_3/4, bram1_12/4, bram1_21/4, bram1_30/4
  debus_dinb1/4(out30) -> bram1_3/5
  debus_web1/4(out6) -> bram1_3/6, bram1_12/6, bram1_21/6, bram1_30/6
  debus_addra1/5(out5) -> bram1_4/1, bram1_13/1, bram1_22/1, bram1_31/1
  debus_dina1/5(out29) -> bram1_4/2
  debus_wea1/5(out5) -> bram1_4/3, bram1_13/3, bram1_22/3, bram1_31/3
  debus_addrb1/5(out5) -> bram1_4/4, bram1_13/4, bram1_22/4, bram1_31/4
  debus_dinb1/5(out29) -> bram1_4/5
  debus_web1/5(out5) -> bram1_4/6, bram1_13/6, bram1_22/6, bram1_31/6
  debus_addra1/6(out4) -> bram1_5/1, bram1_14/1, bram1_23/1, bram1_32/1
  debus_dina1/6(out28) -> bram1_5/2
  debus_wea1/6(out4) -> bram1_5/3, bram1_14/3, bram1_23/3, bram1_32/3
  debus_addrb1/6(out4) -> bram1_5/4, bram1_14/4, bram1_23/4, bram1_32/4
  debus_dinb1/6(out28) -> bram1_5/5
  debus_web1/6(out4) -> bram1_5/6, bram1_14/6, bram1_23/6, bram1_32/6
  debus_addra1/7(out3) -> bram1_6/1, bram1_15/1, bram1_24/1
  debus_dina1/7(out27) -> bram1_6/2
  debus_wea1/7(out3) -> bram1_6/3, bram1_15/3, bram1_24/3
  debus_addrb1/7(out3) -> bram1_6/4, bram1_15/4, bram1_24/4
  debus_dinb1/7(out27) -> bram1_6/5
  debus_web1/7(out3) -> bram1_6/6, bram1_15/6, bram1_24/6
  debus_addra1/8(out2) -> bram1_7/1, bram1_16/1, bram1_25/1
  debus_dina1/8(out26) -> bram1_7/2
  debus_wea1/8(out2) -> bram1_7/3, bram1_16/3, bram1_25/3
  debus_addrb1/8(out2) -> bram1_7/4, bram1_16/4, bram1_25/4
  debus_dinb1/8(out26) -> bram1_7/5
  debus_web1/8(out2) -> bram1_7/6, bram1_16/6, bram1_25/6
  debus_addra1/9(lsb_out1) -> bram1_8/1, bram1_17/1, bram1_26/1
  debus_dina1/9(out25) -> bram1_8/2
  debus_wea1/9(lsb_out1) -> bram1_8/3, bram1_17/3, bram1_26/3
  debus_addrb1/9(lsb_out1) -> bram1_8/4, bram1_17/4, bram1_26/4
  debus_dinb1/9(out25) -> bram1_8/5
  debus_web1/9(lsb_out1) -> bram1_8/6, bram1_17/6, bram1_26/6
  debus_dina1/10(out24) -> bram1_9/2
  debus_dinb1/10(out24) -> bram1_9/5
  debus_dina1/11(out23) -> bram1_10/2
  debus_dinb1/11(out23) -> bram1_10/5
  debus_dina1/12(out22) -> bram1_11/2
  debus_dinb1/12(out22) -> bram1_11/5
  debus_dina1/13(out21) -> bram1_12/2
  debus_dinb1/13(out21) -> bram1_12/5
  debus_dina1/14(out20) -> bram1_13/2
  debus_dinb1/14(out20) -> bram1_13/5
  debus_dina1/15(out19) -> bram1_14/2
  debus_dinb1/15(out19) -> bram1_14/5
  debus_dina1/16(out18) -> bram1_15/2
  debus_dinb1/16(out18) -> bram1_15/5
  debus_dina1/17(out17) -> bram1_16/2
  debus_dinb1/17(out17) -> bram1_16/5
  debus_dina1/18(out16) -> bram1_17/2
  debus_dinb1/18(out16) -> bram1_17/5
  debus_dina1/19(out15) -> bram1_18/2
  debus_dinb1/19(out15) -> bram1_18/5
  debus_dina1/20(out14) -> bram1_19/2
  debus_dinb1/20(out14) -> bram1_19/5
  debus_dina1/21(out13) -> bram1_20/2
  debus_dinb1/21(out13) -> bram1_20/5
  debus_dina1/22(out12) -> bram1_21/2
  debus_dinb1/22(out12) -> bram1_21/5
  debus_dina1/23(out11) -> bram1_22/2
  debus_dinb1/23(out11) -> bram1_22/5
  debus_dina1/24(out10) -> bram1_23/2
  debus_dinb1/24(out10) -> bram1_23/5
  debus_dina1/25(out9) -> bram1_24/2
  debus_dinb1/25(out9) -> bram1_24/5
  debus_dina1/26(out8) -> bram1_25/2
  debus_dinb1/26(out8) -> bram1_25/5
  debus_dina1/27(out7) -> bram1_26/2
  debus_dinb1/27(out7) -> bram1_26/5
  debus_dina1/28(out6) -> bram1_27/2
  debus_dinb1/28(out6) -> bram1_27/5
  debus_dina1/29(out5) -> bram1_28/2
  debus_dinb1/29(out5) -> bram1_28/5
  debus_dina1/30(out4) -> bram1_29/2
  debus_dinb1/30(out4) -> bram1_29/5
  debus_dina1/31(out3) -> bram1_30/2
  debus_dinb1/31(out3) -> bram1_30/5
  debus_dina1/32(out2) -> bram1_31/2
  debus_dinb1/32(out2) -> bram1_31/5
  debus_dina1/33(lsb_out1) -> bram1_32/2
  debus_dinb1/33(lsb_out1) -> bram1_32/5
  bram0_0/1 -> A_bussify0/1(in1)
  bram0_0/2 -> B_bussify0/1(in1)
  bram0_1/1 -> A_bussify0/2(in2)
  bram0_1/2 -> B_bussify0/2(in2)
  bram0_2/1 -> A_bussify0/3(in3)
  bram0_2/2 -> B_bussify0/3(in3)
  bram0_3/1 -> A_bussify0/4(in4)
  bram0_3/2 -> B_bussify0/4(in4)
  bram0_4/1 -> A_bussify0/5(in5)
  bram0_4/2 -> B_bussify0/5(in5)
  bram0_5/1 -> A_bussify0/6(in6)
  bram0_5/2 -> B_bussify0/6(in6)
  bram0_6/1 -> A_bussify0/7(in7)
  bram0_6/2 -> B_bussify0/7(in7)
  bram0_7/1 -> A_bussify0/8(in8)
  bram0_7/2 -> B_bussify0/8(in8)
  bram0_8/1 -> A_bussify0/9(in9)
  bram0_8/2 -> B_bussify0/9(in9)
  bram0_9/1 -> A_bussify0/10(in10)
  bram0_9/2 -> B_bussify0/10(in10)
  bram0_10/1 -> A_bussify0/11(in11)
  bram0_10/2 -> B_bussify0/11(in11)
  bram0_11/1 -> A_bussify0/12(in12)
  bram0_11/2 -> B_bussify0/12(in12)
  bram0_12/1 -> A_bussify0/13(in13)
  bram0_12/2 -> B_bussify0/13(in13)
  bram0_13/1 -> A_bussify0/14(in14)
  bram0_13/2 -> B_bussify0/14(in14)
  bram0_14/1 -> A_bussify0/15(in15)
  bram0_14/2 -> B_bussify0/15(in15)
  bram0_15/1 -> A_bussify0/16(in16)
  bram0_15/2 -> B_bussify0/16(in16)
  bram0_16/1 -> A_bussify0/17(in17)
  bram0_16/2 -> B_bussify0/17(in17)
  bram0_17/1 -> A_bussify0/18(in18)
  bram0_17/2 -> B_bussify0/18(in18)
  bram0_18/1 -> A_bussify0/19(in19)
  bram0_18/2 -> B_bussify0/19(in19)
  bram0_19/1 -> A_bussify0/20(in20)
  bram0_19/2 -> B_bussify0/20(in20)
  bram0_20/1 -> A_bussify0/21(in21)
  bram0_20/2 -> B_bussify0/21(in21)
  bram0_21/1 -> A_bussify0/22(in22)
  bram0_21/2 -> B_bussify0/22(in22)
  bram0_22/1 -> A_bussify0/23(in23)
  bram0_22/2 -> B_bussify0/23(in23)
  bram0_23/1 -> A_bussify0/24(in24)
  bram0_23/2 -> B_bussify0/24(in24)
  bram0_24/1 -> A_bussify0/25(in25)
  bram0_24/2 -> B_bussify0/25(in25)
  bram0_25/1 -> A_bussify0/26(in26)
  bram0_25/2 -> B_bussify0/26(in26)
  bram0_26/1 -> A_bussify0/27(in27)
  bram0_26/2 -> B_bussify0/27(in27)
  bram0_27/1 -> A_bussify0/28(in28)
  bram0_27/2 -> B_bussify0/28(in28)
  bram0_28/1 -> A_bussify0/29(in29)
  bram0_28/2 -> B_bussify0/29(in29)
  bram0_29/1 -> A_bussify0/30(in30)
  bram0_29/2 -> B_bussify0/30(in30)
  bram0_30/1 -> A_bussify0/31(in31)
  bram0_30/2 -> B_bussify0/31(in31)
  bram0_31/1 -> A_bussify0/32(in32)
  bram0_31/2 -> B_bussify0/32(in32)
  bram0_32/1 -> A_bussify0/33(in33)
  bram0_32/2 -> B_bussify0/33(in33)
  bram1_0/1 -> A_bussify1/1(in1)
  bram1_0/2 -> B_bussify1/1(in1)
  bram1_1/1 -> A_bussify1/2(in2)
  bram1_1/2 -> B_bussify1/2(in2)
  bram1_2/1 -> A_bussify1/3(in3)
  bram1_2/2 -> B_bussify1/3(in3)
  bram1_3/1 -> A_bussify1/4(in4)
  bram1_3/2 -> B_bussify1/4(in4)
  bram1_4/1 -> A_bussify1/5(in5)
  bram1_4/2 -> B_bussify1/5(in5)
  bram1_5/1 -> A_bussify1/6(in6)
  bram1_5/2 -> B_bussify1/6(in6)
  bram1_6/1 -> A_bussify1/7(in7)
  bram1_6/2 -> B_bussify1/7(in7)
  bram1_7/1 -> A_bussify1/8(in8)
  bram1_7/2 -> B_bussify1/8(in8)
  bram1_8/1 -> A_bussify1/9(in9)
  bram1_8/2 -> B_bussify1/9(in9)
  bram1_9/1 -> A_bussify1/10(in10)
  bram1_9/2 -> B_bussify1/10(in10)
  bram1_10/1 -> A_bussify1/11(in11)
  bram1_10/2 -> B_bussify1/11(in11)
  bram1_11/1 -> A_bussify1/12(in12)
  bram1_11/2 -> B_bussify1/12(in12)
  bram1_12/1 -> A_bussify1/13(in13)
  bram1_12/2 -> B_bussify1/13(in13)
  bram1_13/1 -> A_bussify1/14(in14)
  bram1_13/2 -> B_bussify1/14(in14)
  bram1_14/1 -> A_bussify1/15(in15)
  bram1_14/2 -> B_bussify1/15(in15)
  bram1_15/1 -> A_bussify1/16(in16)
  bram1_15/2 -> B_bussify1/16(in16)
  bram1_16/1 -> A_bussify1/17(in17)
  bram1_16/2 -> B_bussify1/17(in17)
  bram1_17/1 -> A_bussify1/18(in18)
  bram1_17/2 -> B_bussify1/18(in18)
  bram1_18/1 -> A_bussify1/19(in19)
  bram1_18/2 -> B_bussify1/19(in19)
  bram1_19/1 -> A_bussify1/20(in20)
  bram1_19/2 -> B_bussify1/20(in20)
  bram1_20/1 -> A_bussify1/21(in21)
  bram1_20/2 -> B_bussify1/21(in21)
  bram1_21/1 -> A_bussify1/22(in22)
  bram1_21/2 -> B_bussify1/22(in22)
  bram1_22/1 -> A_bussify1/23(in23)
  bram1_22/2 -> B_bussify1/23(in23)
  bram1_23/1 -> A_bussify1/24(in24)
  bram1_23/2 -> B_bussify1/24(in24)
  bram1_24/1 -> A_bussify1/25(in25)
  bram1_24/2 -> B_bussify1/25(in25)
  bram1_25/1 -> A_bussify1/26(in26)
  bram1_25/2 -> B_bussify1/26(in26)
  bram1_26/1 -> A_bussify1/27(in27)
  bram1_26/2 -> B_bussify1/27(in27)
  bram1_27/1 -> A_bussify1/28(in28)
  bram1_27/2 -> B_bussify1/28(in28)
  bram1_28/1 -> A_bussify1/29(in29)
  bram1_28/2 -> B_bussify1/29(in29)
  bram1_29/1 -> A_bussify1/30(in30)
  bram1_29/2 -> B_bussify1/30(in30)
  bram1_30/1 -> A_bussify1/31(in31)
  bram1_30/2 -> B_bussify1/31(in31)
  bram1_31/1 -> A_bussify1/32(in32)
  bram1_31/2 -> B_bussify1/32(in32)
  bram1_32/1 -> A_bussify1/33(in33)
  bram1_32/2 -> B_bussify1/33(in33)
  damsbs/1 -> mux_A/1
  dbmsbs/1 -> mux_B/1
  A_bussify0/1(bus_out) -> mux_A/2
  B_bussify0/1(bus_out) -> mux_B/2
  A_bussify1/1(bus_out) -> mux_A/3
  B_bussify1/1(bus_out) -> mux_B/3
  mux_A/1 -> A/1
  mux_B/1 -> B/1

== system deep_bram/bus_expand ==
  bus_in : Inport
  reinterpret{1..4} (4 alike) : xbsIndex_r4/Reinterpret  force_arith_type=on  arith_type=Unsigned  force_bin_pt=on  bin_pt=0  block_type=reinterpret
  slice1 : xbsIndex_r4/Slice  nbits=33  boolean_output=off  mode=Upper Bit Location + Width  bit1=-99  base1=MSB of Input  bit0=0  base0=LSB of Input  dbl_ovrd=off  block_type=slice
  slice2 : xbsIndex_r4/Slice  nbits=33  boolean_output=off  mode=Upper Bit Location + Width  bit1=-66  base1=MSB of Input  bit0=0  base0=LSB of Input  dbl_ovrd=off  block_type=slice
  slice3 : xbsIndex_r4/Slice  nbits=33  boolean_output=off  mode=Upper Bit Location + Width  bit1=-33  base1=MSB of Input  bit0=0  base0=LSB of Input  dbl_ovrd=off  block_type=slice
  slice4 : xbsIndex_r4/Slice  nbits=33  boolean_output=off  mode=Upper Bit Location + Width  bit1=0  base1=MSB of Input  bit0=0  base0=LSB of Input  dbl_ovrd=off  block_type=slice
  msb_out4 : Outport
  out3 : Outport  Port=2
  out2 : Outport  Port=3
  lsb_out1 : Outport  Port=4
  wires:
  bus_in/1 -> slice4/1, slice3/1, slice2/1, slice1/1
  slice4/1 -> reinterpret4/1
  reinterpret4/1 -> msb_out4/1
  slice3/1 -> reinterpret3/1
  reinterpret3/1 -> out3/1
  slice2/1 -> reinterpret2/1
  reinterpret2/1 -> out2/1
  slice1/1 -> reinterpret1/1
  reinterpret1/1 -> lsb_out1/1
